simulink model "dynmodel_KUKA_cascade_task_v2014"  (R2015a)
settings: Solver=ode45  StartTime=0.0  StopTime=10  RelTol=1e-3
values from neighbouring files (symbols this model uses):
  d2 = 0.033    [dynamique_youbot.m]    (also in dynamique_youbot_VersaoSemPI.m; dynamique_youbot_test.m; inverse_geometric_model.m)
  d3 = 0.155    [dynamique_youbot.m]    (also in dynamique_youbot_VersaoSemPI.m; dynamique_youbot_test.m; inverse_geometric_model.m)
  d4 = 0.135    [dynamique_youbot.m]    (also in dynamique_youbot_VersaoSemPI.m; dynamique_youbot_test.m; inverse_geometric_model.m)
  lend = 0.218    [dynamique_youbot.m]    (also in dynamique_youbot_VersaoSemPI.m; dynamique_youbot_test.m; inverse_geometric_model.m)
  th_DHM = -th_KUKA + offset    [dynamique_youbot.m]    (also in dynamique_youbot_VersaoSemPI.m; dynamique_youbot_test.m)
undefined symbols (not defined in the file or in its folder): trajectory, vitesse
libraries: simulink x1
settings Model: CovModelRefEnable=off  Creator=dejesusrodri_tia  LastModifiedBy=Karoline
settings DataIOCC: LimitDataPoints=off  SaveFormat=StructureWithTime
settings HardwareCC: ProdBitPerPointer=64  ProdLargestAtomicFloat=Float  ProdIntDivRoundTo=Zero  ProdEndianess=LittleEndian  ProdHWDeviceType=Specified
settings ModelReferenceCC: PropagateSignalLabelsOutOfModel=on

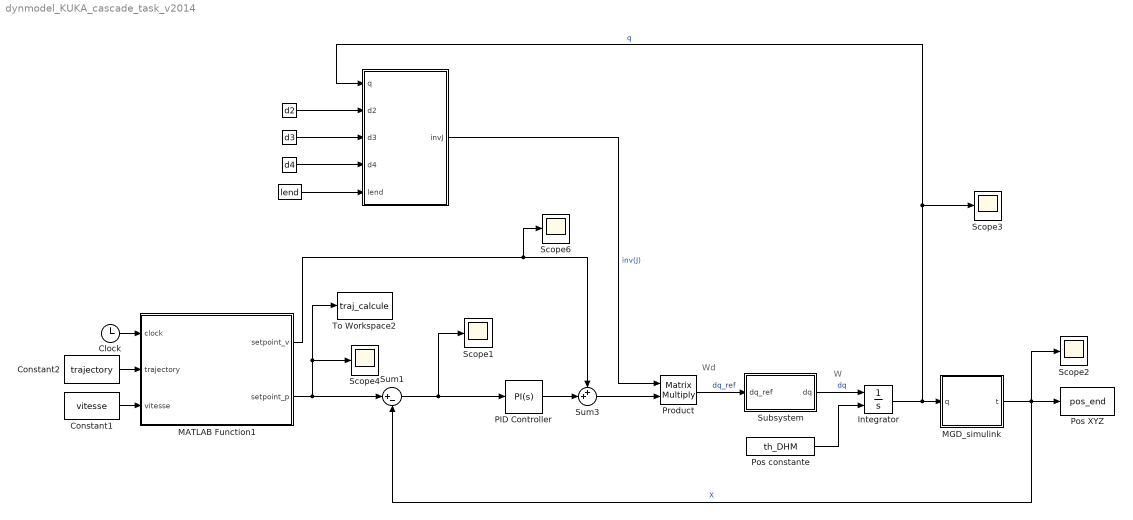
== system dynmodel_KUKA_cascade_task_v2014 ==
  note: Wd
  note: W
  " " : MATLAB Function  TreatAsAtomicUnit=on
  " " : Constant  Value=d3
  " " : Constant  Value=d2  OutDataTypeStr=double
  " " : Constant  Value=d4
  "     " : Constant  Value=lend
  Clock : Clock
  Constant1 : Constant  Value=vitesse  VectorParams1D=off
  Constant2 : Constant  Value=trajectory  VectorParams1D=off
  Integrator : Integrator  InitialConditionSource=external  InitialCondition=th_DHM
  MATLAB Function1 : MATLAB Function  TreatAsAtomicUnit=on
  MGD_simulink : MATLAB Function  TreatAsAtomicUnit=on
  PID Controller : simulink/Continuous/PID Controller  Controller=PI  TimeDomain=Continuous-time  SampleTime=-1  IntegratorMethod=Forward Euler  FilterMethod=Forward Euler  Form=Parallel  UseFilter=on  ControllerParametersSource=internal  P=1  I=0  D=0  N=100  InitialConditionSource=internal  InitialConditionForIntegrator=0  InitialConditionForFilter=0  ExternalReset=none  LimitOutput=off  UpperSaturationLimit=inf  LowerSaturationLimit=-inf  LinearizeAsGain=on  AntiWindupMode=none  Kb=1  TrackingMode=off  Kt=1  PParamMin=[]  PParamMax=[]  IParamMin=[]  IParamMax=[]  DParamMin=[]  DParamMax=[]  NParamMin=[]  NParamMax=[]  KbParamMin=[]  KbParamMax=[]  KtParamMin=[]  KtParamMax=[]  POutMin=[]  POutMax=[]  IOutMin=[]  IOutMax=[]  DOutMin=[]  DOutMax=[]  NOutMin=[]  NOutMax=[]  KbOutMin=[]  KbOutMax=[]  KtOutMin=[]  KtOutMax=[]  IntegratorOutMin=[]  IntegratorOutMax=[]  FilterOutMin=[]  FilterOutMax=[]  SumOutMin=[]  SumOutMax=[]  SumI1OutMin=[]  SumI1OutMax=[]  SumI2OutMin=[]  SumI2OutMax=[]  SumI3OutMin=[]  SumI3OutMax=[]  SumDOutMin=[]  SumDOutMax=[]  SaturationOutMin=[]  SaturationOutMax=[]  IntegratorContinuousStateAttributes=''  IntegratorStateMustResolveToSignalObject=off  IntegratorRTWStateStorageClass=Auto  FilterContinuousStateAttributes=''  FilterStateMustResolveToSignalObject=off  FilterRTWStateStorageClass=Auto  DifferentiatorICPrevScaledInput=0  DifferentiatorOutMin=[]  DifferentiatorOutMax=[]
  Pos XYZ : ToWorkspace  VariableName=pos_end  SaveFormat=Structure With Time  SampleTime=-1
  Pos constante : Constant  Value=th_DHM  VectorParams1D=off
  Product : Product  Multiplication=Matrix(*)
  Scope{1..4,6} (5 alike) : Scope
      Scope1 settings: YMin=-0.70507  YMax=1.07714  SaveName=ScopeData2
      Scope2 settings: ShowLegends=on  YMin=-0.66443  YMax=0.80147  SaveName=ScopeData5
      Scope3 settings: ShowLegends=on  YMin=-0.04314  YMax=0.03878
      Scope4 settings: YMin=-0.05587  YMax=0.50287
      Scope6 settings: YMin=-0.05587  YMax=0.50287  SaveName=ScopeData2
  Subsystem : Subsystem
  Sum1 : Sum  Inputs=|+-
  Sum3 : Sum  Inputs=++|
  To Workspace2 : ToWorkspace  VariableName=traj_calcule  SampleTime=-1
  wires:
  " "/1 -> " "/2(d2)
  " "/1 -> " "/3(d3)
  " "/1 -> " "/4(d4)
  "     "/1 -> " "/5(lend)
  MGD_simulink/1(t) -> Scope2/1, Sum1/2, Pos XYZ/1  "X"
  Sum3/1 -> Product/2
  " "/1(invJ) -> Product/1  "inv(J)"
  Subsystem/1(dq) -> Integrator/1  "dq"
  Product/1 -> Subsystem/1(dq_ref)  "dq_ref"
  Integrator/1 -> MGD_simulink/1(q), " "/1(q), Scope3/1  "q"
  Pos constante/1 -> Integrator/2
  MATLAB Function1/2(setpoint_p) -> Sum1/1, To Workspace2/1, Scope4/1
  Constant2/1 -> MATLAB Function1/2(trajectory)
  Sum1/1 -> Scope1/1, PID Controller/1
  PID Controller/1 -> Sum3/2
  Clock/1 -> MATLAB Function1/1(clock)
  Constant1/1 -> MATLAB Function1/3(vitesse)
  MATLAB Function1/1(setpoint_v) -> Scope6/1, Sum3/1

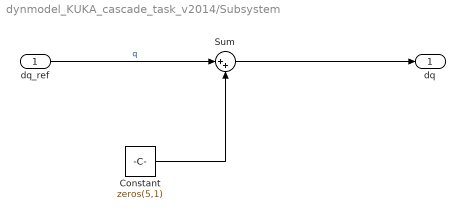
== system dynmodel_KUKA_cascade_task_v2014/Subsystem ==
  dq_ref : Inport
  Constant : Constant  Value=zeros(5,1)
  Sum : Sum  Inputs=|++
  dq : Outport
  wires:
  dq_ref/1 -> Sum/1  "q"
  Sum/1 -> dq/1
  Constant/1 -> Sum/2

== matlab function dynmodel_KUKA_cascade_task_v2014/MGD_simulink ==
  data: q input; t output size=3; param parameter
function t  = fcn(q,param)

th1 = q(1);
th2 = q(2);
th3 = q(3);
th4 = q(4);

% introduction des paramètres
d1=param.d1;
r1=param.r1;
d2=param.d2;
d3=param.d3;
d4=param.d4;
lend = param.lend;

t = MGD_end(d1,d2,d3,d4,lend,r1,th1,th2,th3,th4);

== matlab function dynmodel_KUKA_cascade_task_v2014/  ==
  data: invJ output; q input; d2 input; d3 input; d4 input; lend input
function invJ   = vitesse_lin(q,d2,d3,d4,lend)

th1 = q(1);
th2 = q(2);
th3 = q(3);
th4 = q(4);

J = Jacobian_youbot(d2,d3,d4,lend,th1,th2,th3,th4);

% Outputs
invJ = pinv(J);

end

== matlab function dynmodel_KUKA_cascade_task_v2014/MATLAB Function1 ==
  data: setpoint_v output; clock input; setpoint_p output; trajectory input; vitesse input
function [setpoint_v, setpoint_p]  = select_element(clock,trajectory,vitesse)

if (clock*1000) < size(trajectory,2)
    setpoint_p = trajectory(:,floor((clock+0.001)*1000));
    setpoint_v = vitesse(:,floor((clock+0.001)*1000));
else
    setpoint_p = trajectory(:,size(trajectory,2));
    setpoint_v = vitesse(:,size(trajectory,2));
end

end
